simulink model "rlSimplePendulumModel"  (R2018a)
settings: Solver=ode45  StartTime=0.0  StopTime=Tf  RelTol=1e-5  AbsTol=1e-6
model workspace (MAT data in the model file):
  I = 0
  c = 0
  g = 9.81
  l = 1
  m = 1
  max_tau = 2
  theta0 = 0
  theta_dot0 = 0
libraries: rllib x1
settings Model: Creator=The MathWorks, Inc.  LastModifiedBy=hhq
settings SolverCC: AutoScaleAbsTol=off
settings DataIOCC: LimitDataPoints=on  SaveFormat=Array  SaveState=on  ReturnWorkspaceOutputs=on
settings OptimizationCC: BlockReduction=off  BooleanDataType=off  LifeSpan=inf
settings DebuggingCC: SaveWithParameterizedLinksMsg=none  SignalResolutionControl=TryResolveAllWithWarning  SFUnexpectedBacktrackingDiag=warning  SFNoUnconditionalDefaultTransitionDiag=warning  SFExecutionAtInitializationDiag=none
settings HardwareCC: ProdBitPerPointer=32  ProdBitPerSizeT=32  ProdBitPerPtrDiffT=32  ProdLargestAtomicFloat=None  ProdIntDivRoundTo=Undefined  ProdEndianess=Unspecified  ProdWordSize=32  ProdHWDeviceType=32-bit Generic  TargetUnknown=on
settings ModelReferenceCC: PropagateSignalLabelsOutOfModel=off
settings CodeAppCC: StateflowObjectComments=on
settings GRTTargetCC: TargetLangStandard=C89/C90 (ANSI)  GeneratePreprocessorConditionals=Disable all
settings ConfigComp: CovMetricSettings=dw  CovHtmlReporting=on  CovSaveCumulativeToWorkspaceVar=on  CovSaveSingleToWorkspaceVar=on  CovExternalEMLEnable=off

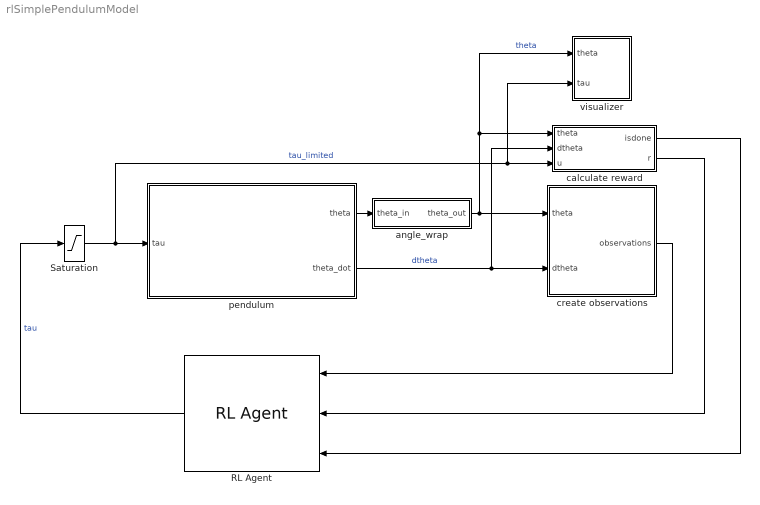
== system rlSimplePendulumModel ==
  RL Agent : rllib/RL Agent  Agent=agent  ProvideReward=on  ProvideIsDone=on  ProvideCumRwd=off  TreatAsDirectFeedthrough=on  CollectLoggedSignals=on  CollectModelStates=on
      settings: SourceProductName=The database C:\Users\ddavis\AppData\Roaming\MathWorks\MATLAB\R2018b\slblocks_master.db is locked, or a table in the database is locked. (database is locked)
  Saturation : Saturate  UpperLimit=max_tau  LowerLimit=-max_tau
  angle_wrap : Subsystem
  calculate reward : Subsystem
  create observations : Subsystem  Variant=on  VariantControl=Variant1  OverrideUsingVariant=sincos  mask{ThetaObservationHandling=sincos}
      mask prompts: ThetaObservationHandling "Select how theta is treated in the observation vector"
      mask init:
      | simulationStatus = get_param(bdroot,'SimulationStatus');
      | 
      | % The active variant can only be modified at edit-time or very early during
      | % the simulink compile stage. 
      | 
      | choice = get_param(gcb,'ThetaObservationHandling');
      | oldVariant = get_param(gcb,'OverrideUsingVariant');
      | 
      | switch choice
      |     case 'theta'
      |     case 'sincos'
      |     otherwise
      |         error('%s is not supported',choice)
      | end
      | set_param(gcb,'OverrideUsingVariant',choice);
      mask TypeOptions ThetaObservationHandling: theta | sincos
  pendulum : Subsystem
  visualizer : Subsystem
  wires:
  pendulum/2(theta_dot) -> calculate reward/2(dtheta), create observations/2("dtheta ")  "dtheta"
  pendulum/1(theta) -> angle_wrap/1(theta_in)
  angle_wrap/1(theta_out) -> visualizer/1(theta), calculate reward/1(theta), create observations/1("theta ")  "theta"
  calculate reward/2(r) -> RL Agent/2
  calculate reward/1(isdone) -> RL Agent/3
  RL Agent/1 -> Saturation/1  "tau"
  Saturation/1 -> visualizer/2(tau), calculate reward/3(u), pendulum/1(tau)  "tau_limited"
  create observations/1(" observations") -> RL Agent/1

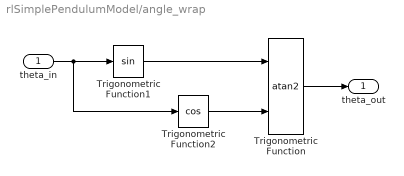
== system rlSimplePendulumModel/angle_wrap ==
  theta_in : Inport
  Trigonometric Function : Trigonometry  Operator=atan2
  Trigonometric Function1 : Trigonometry
  Trigonometric Function2 : Trigonometry  Operator=cos
  theta_out : Outport
  wires:
  theta_in/1 -> Trigonometric Function2/1, Trigonometric Function1/1
  Trigonometric Function/1 -> theta_out/1
  Trigonometric Function1/1 -> Trigonometric Function/1
  Trigonometric Function2/1 -> Trigonometric Function/2

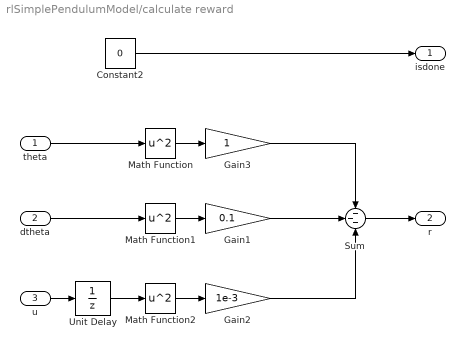
== system rlSimplePendulumModel/calculate reward ==
  theta : Inport
  dtheta : Inport  Port=2
  u : Inport  Port=3
  Constant2 : Constant  Value=0
  Gain1 : Gain  Gain=0.1
  Gain2 : Gain  Gain=1e-3
  Gain3 : Gain
  Math Function : Math  Operator=square  SaturateOnIntegerOverflow=on
  Math Function1 : Math  Operator=square  SaturateOnIntegerOverflow=on
  Math Function2 : Math  Operator=square  SaturateOnIntegerOverflow=on
  Sum : Sum  Inputs=---
  Unit Delay : UnitDelay  SampleTime=-1  HasFrameUpgradeWarning=on
  isdone : Outport
  r : Outport  Port=2
  wires:
  Constant2/1 -> isdone/1
  theta/1 -> Math Function/1
  dtheta/1 -> Math Function1/1
  u/1 -> Unit Delay/1
  Sum/1 -> r/1
  Math Function/1 -> Gain3/1
  Math Function1/1 -> Gain1/1
  Math Function2/1 -> Gain2/1
  Gain2/1 -> Sum/3
  Gain1/1 -> Sum/2
  Gain3/1 -> Sum/1
  Unit Delay/1 -> Math Function2/1

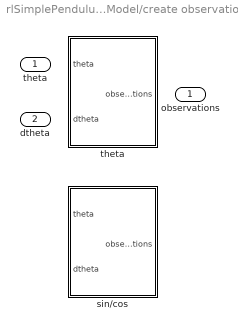
== system rlSimplePendulumModel/create observations ==
  "theta " : Inport
  "dtheta " : Inport  Port=2
  sin/cos : Subsystem  VariantControl=sincos
  theta : Subsystem  VariantControl=theta
  " observations" : Outport

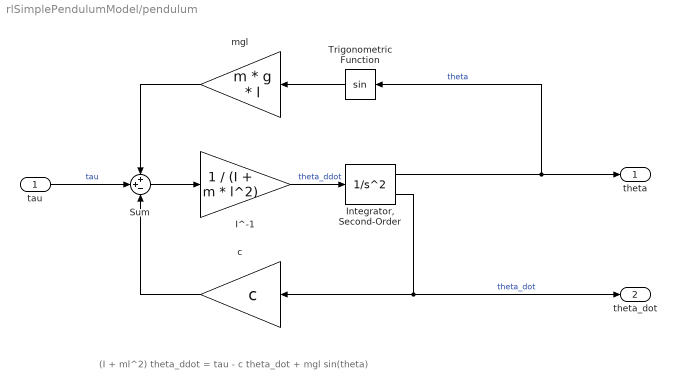
== system rlSimplePendulumModel/pendulum ==
  note: (I + ml^2) theta_ddot = tau - c theta_dot + mgl sin(theta)
  tau : Inport
  I^-1 : Gain  Gain=1 / (I + m * l^2)
  "Integrator, Second-Order" : SecondOrderIntegrator  ICX=theta0  UpperLimitX=1  LowerLimitX=0  StateNameX='theta'  ICDXDT=theta_dot0  StateNameDXDT='theta_dot'
  Sum : Sum  Inputs=++-
  Trigonometric Function : Trigonometry
  c : Gain  Gain=c
  mgl : Gain  Gain=m * g * l
  theta : Outport
  theta_dot : Outport  Port=2
  wires:
  mgl/1 -> Sum/1
  c/1 -> Sum/3
  Trigonometric Function/1 -> mgl/1
  Sum/1 -> I^-1/1
  "Integrator, Second-Order"/1 -> theta/1, Trigonometric Function/1  "theta"
  I^-1/1 -> "Integrator, Second-Order"/1  "theta_ddot"
  "Integrator, Second-Order"/2 -> c/1, theta_dot/1  "theta_dot"
  tau/1 -> Sum/2  "tau"

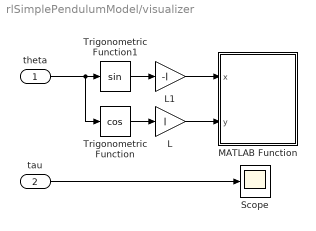
== system rlSimplePendulumModel/visualizer ==
  theta : Inport
  tau : Inport  Port=2
  L : Gain  Gain=l
  L1 : Gain  Gain=-l
  MATLAB Function : MATLAB Function  TreatAsAtomicUnit=on
  Scope : Scope
  Trigonometric Function : Trigonometry  Operator=cos
  Trigonometric Function1 : Trigonometry
  wires:
  theta/1 -> Trigonometric Function/1, Trigonometric Function1/1
  L1/1 -> MATLAB Function/1(x)
  Trigonometric Function/1 -> L/1
  L/1 -> MATLAB Function/2(y)
  Trigonometric Function1/1 -> L1/1
  tau/1 -> Scope/1

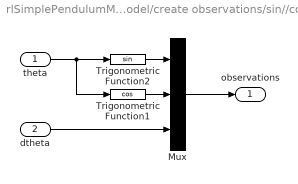
== system rlSimplePendulumModel/create observations/sin//cos ==
  theta : Inport
  dtheta : Inport  Port=2
  Mux : Mux  Inputs=3
  Trigonometric Function1 : Trigonometry  Operator=cos
  Trigonometric Function2 : Trigonometry
  observations : Outport
  wires:
  theta/1 -> Trigonometric Function1/1, Trigonometric Function2/1
  Mux/1 -> observations/1
  dtheta/1 -> Mux/3
  Trigonometric Function2/1 -> Mux/1
  Trigonometric Function1/1 -> Mux/2

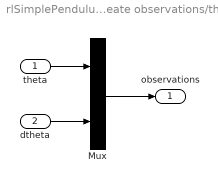
== system rlSimplePendulumModel/create observations/theta ==
  theta : Inport
  dtheta : Inport  Port=2
  Mux : Mux  Inputs=2
  observations : Outport
  wires:
  dtheta/1 -> Mux/2
  Mux/1 -> observations/1
  theta/1 -> Mux/1

== matlab function rlSimplePendulumModel/visualizer/MATLAB Function ==
  settings: updateMethod=DISCRETE
  data: x input; y input
function plotPend(x,y)
% plot the simple pendulum
coder.extrinsic('rl.env.viz.plotSimplePendulum');
rl.env.viz.plotSimplePendulum(x,y);
